simulink model "motor"  (R2020b)
settings: Solver=VariableStepAuto  StartTime=0.0  StopTime=10.0  RelTol=1e-3
settings Model: Creator=ericb  LastModifiedBy=ericb

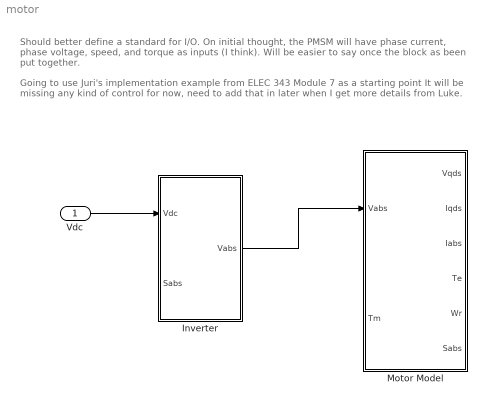
== system motor ==
  note: Going to use Juri's implementation example from ELEC 343 Module 7 as a starting point
      | It will be missing any kind of control for now, need to add that in later when I get more details from Luke.
  note: Should better define a standard for I/O. On initial thought, the PMSM will have phase current, phase voltage, speed, and torque as inputs (I think). Will be easier to say once the block as been put together.
  Vdc : Inport
  Inverter : Subsystem
  Motor Model : Subsystem
  wires:
  Inverter/1(Vabs) -> Motor Model/1(Vabs)
  Vdc/1 -> Inverter/1(Vdc)

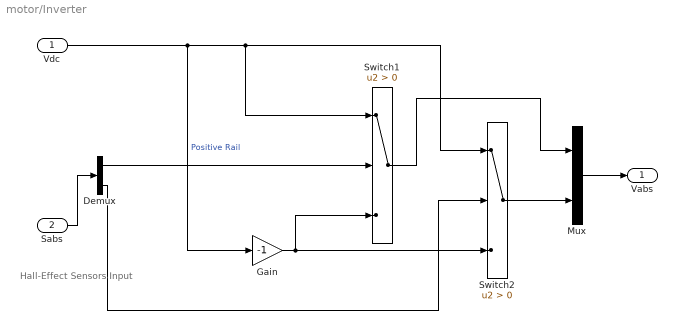
== system motor/Inverter ==
  note: Hall-Effect Sensors Input
  Vdc : Inport
  Sabs : Inport  Port=2
  Demux : Demux  Outputs=2
  Gain : Gain  Gain=-1
  Mux : Mux  Inputs=2
  Switch1 : Switch  Criteria=u2 > Threshold
  Switch2 : Switch  Criteria=u2 > Threshold
  Vabs : Outport
  wires:
  Mux/1 -> Vabs/1
  Sabs/1 -> Demux/1
  Vdc/1 -> Switch2/1, Switch1/1, Gain/1  "Positive Rail"
  Switch2/1 -> Mux/2
  Demux/2 -> Switch2/2
  Gain/1 -> Switch1/3, Switch2/3
  Demux/1 -> Switch1/2
  Switch1/1 -> Mux/1

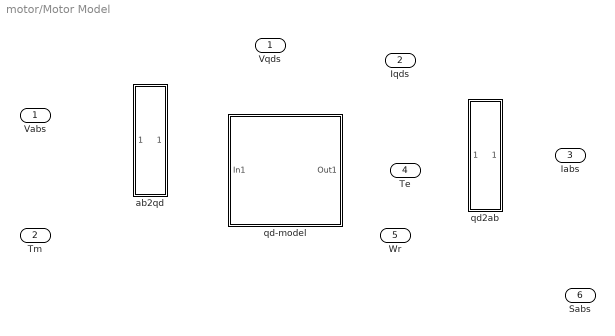
== system motor/Motor Model ==
  Vabs : Inport
  Tm : Inport  Port=2
  ab2qd : Subsystem
  qd-model : Subsystem
  qd2ab : Subsystem
  Vqds : Outport
  Iqds : Outport  Port=2
  Iabs : Outport  Port=3
  Te : Outport  Port=4
  Wr : Outport  Port=5
  Sabs : Outport  Port=6

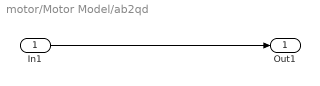
== system motor/Motor Model/ab2qd ==
  In1 : Inport
  Out1 : Outport
  wires:
  In1/1 -> Out1/1

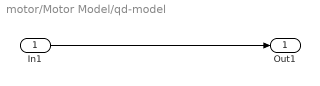
== system motor/Motor Model/qd-model ==
  In1 : Inport
  Out1 : Outport
  wires:
  In1/1 -> Out1/1

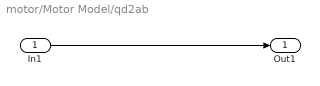
== system motor/Motor Model/qd2ab ==
  In1 : Inport
  Out1 : Outport
  wires:
  In1/1 -> Out1/1
